simulink model "OnePointMassSim"  (R2020b)
settings: Solver=VariableStepAuto  StartTime=0.0  StopTime=100  RelTol=1e-3
undefined symbols (not defined in the file): A, alpha_stat, B, C, my_stat, sigmaf_stat, T_start, X_init
settings Model: Creator=teteu  LastModifiedBy=teteu

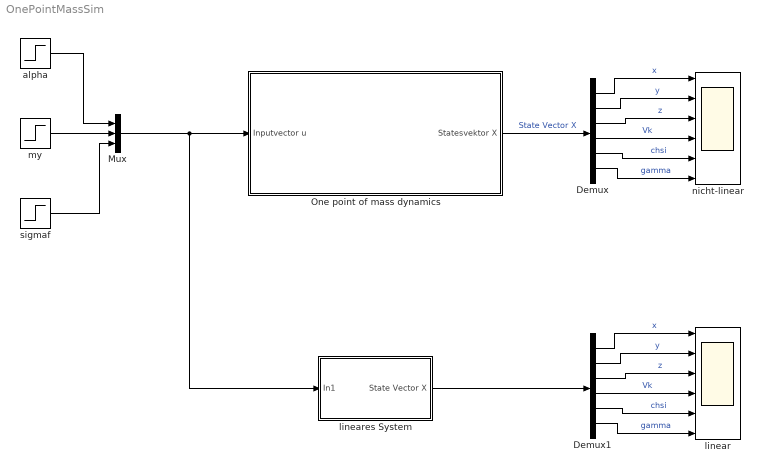
== system OnePointMassSim ==
  Demux : Demux  Outputs=6
  Demux1 : Demux  Outputs=6
  Mux : Mux  Inputs=3
  One point of mass dynamics : Subsystem
      mask Display: image('F-16 Bild.jpg'); % Use "Edit Image" on toolstrip to change.
  alpha : Step  Time=T_start  After=alpha_stat  SampleTime=0
  linear : Scope  NumInputPorts=6
  lineares System : Subsystem
  my : Step  Time=T_start  After=my_stat  SampleTime=sigmaf_stat
  nicht-linear : Scope  NumInputPorts=6
  sigmaf : Step  SampleTime=0
  wires:
  Mux/1 -> lineares System/1(In1), One point of mass dynamics/1(Inputvector u)
  alpha/1 -> Mux/1
  my/1 -> Mux/2
  sigmaf/1 -> Mux/3
  One point of mass dynamics/1(Statesvektor X) -> Demux/1  "State Vector X"
  Demux/1 -> nicht-linear/1  "x"
  Demux/2 -> nicht-linear/2  "y"
  Demux/3 -> nicht-linear/3  "z"
  Demux/4 -> nicht-linear/4  "Vk"
  Demux/5 -> nicht-linear/5  "chsi"
  Demux/6 -> nicht-linear/6  "gamma"
  Demux1/1 -> linear/1  "x"
  Demux1/5 -> linear/5  "chsi"
  Demux1/6 -> linear/6  "gamma"
  Demux1/4 -> linear/4  "Vk"
  Demux1/3 -> linear/3  "z"
  Demux1/2 -> linear/2  "y"
  lineares System/1(State Vector X) -> Demux1/1

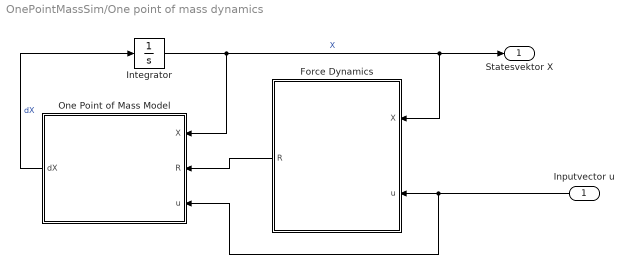
== system OnePointMassSim/One point of mass dynamics ==
  Inputvector u : Inport
  Force Dynamics : MATLAB Function  TreatAsAtomicUnit=on
  Integrator : Integrator  InitialCondition=X_init
  One Point of Mass Model : MATLAB Function  TreatAsAtomicUnit=on
  Statesvektor X : Outport
  wires:
  Integrator/1 -> Force Dynamics/1(X), Statesvektor X/1, One Point of Mass Model/1(X)  "X"
  Inputvector u/1 -> One Point of Mass Model/3(u), Force Dynamics/2(u)
  One Point of Mass Model/1(dX) -> Integrator/1  "dX"
  Force Dynamics/1(R) -> One Point of Mass Model/2(R)

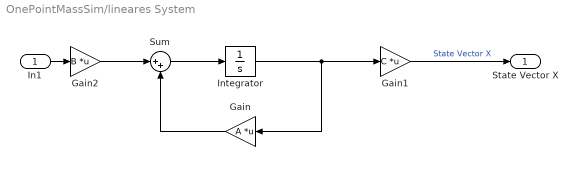
== system OnePointMassSim/lineares System ==
  In1 : Inport
  Gain : Gain  Gain=A  Multiplication=Matrix(K*u)
  Gain1 : Gain  Gain=C  Multiplication=Matrix(K*u)
  Gain2 : Gain  Gain=B  Multiplication=Matrix(K*u)
  Integrator : Integrator  InitialCondition=X_init
  Sum : Sum  Inputs=|++
  State Vector X : Outport
  wires:
  In1/1 -> Gain2/1
  Integrator/1 -> Gain/1, Gain1/1
  Gain/1 -> Sum/2
  Sum/1 -> Integrator/1
  Gain2/1 -> Sum/1
  Gain1/1 -> State Vector X/1  "State Vector X"

== matlab function OnePointMassSim/One point of mass dynamics/Force Dynamics ==
  data: X input; u input; R output; globalConstants parameter
function R = fcn(X,u,globalConstants)
%R Forces involved in the dynamics
% u input of the System
% X States Vector
alpha = u(1); %Angle of Attack 
sigmaf = u(3); %Schubhebstellung
Vk = X(4); %Bahngeschwindigkeit



%Global Parameters 
CA_0 = globalConstants.CA_0;
CA_alpha = globalConstants.CA_alpha;
kw = globalConstants.kw;
F_max = globalConstants.F_max;
rho = globalConstants.rho;
S = globalConstants.S;
%Beiwerte
q = 0.5*rho*Vk^2; %Staudruck (back pressure)
CA = CA_0 +alpha*CA_alpha;
CW = kw*CA^2;

% Force equations 
F =F_max*sin(sigmaf);
A = q*S*CA;
W = q*S*CW;
Q = 0;

R = zeros(4,1);
R(1) = F;
R(2) = -W;
R(3) = Q;
R(4) = -A;

== matlab function OnePointMassSim/One point of mass dynamics/One Point of Mass Model ==
  data: X input; R input; u input; dX output; globalConstants parameter
function dX = fcn(X,R,u,globalConstants)
%dX Derivatives of the States
%X Statesvector: x,y,z (geodastic reference frame), Vk,chsi, gamma
%Ra Forcer F, A, W 
%u Inputvector 
Vk = X(4); %Absolute Value of the Speed in "Bahnsystem" Reference Frame
chsi = X(5); %Bahnazimut (azimuth)
gamma = X(6); %Bahnneigungswinkel (inclination angle)
F = R(1); %Schubkraft (Thrust)
W = -R(2);
A = -R(4);
alpha = u(1); %Angle of Attack
my = u(2);
%Constants
g = globalConstants.g; %Gravity
m = globalConstants.m; % Mass
%Dynamics
dx = Vk*cos(chsi)*cos(gamma);
dy = Vk*sin(chsi)*cos(gamma);
dz = - Vk*sin(gamma);
dVk = (F*cos(alpha)-W)/m - g*sin(gamma);
dchsi = 1/(m*Vk*cos(gamma))*(A*sin(my)+ F*sin(my)*sin(alpha));
dgamma = (cos(my))/(Vk*m)*(A+F*sin(alpha))-g*cos(gamma)/Vk;

%Output Vector
dX = zeros(6,1);
dX(1) = dx;
dX(2) = dy;
dX(3) = dz;
dX(4) = dVk;
dX(5) = dchsi;
dX(6) = dgamma;
